simulink model "lander"  (R2016b)
settings: Solver=FixedStepDiscrete  StartTime=0.0  StopTime=10  FixedStep=0.1  RelTol=1e-3
undefined symbols (not defined in the file): AtmosphereDensityRate, DiscIntNeverNeededParam, GravityConstant, InitialHeight, InitialVelocity, Mass, ProcessNoise
settings Model: Creator=csax  LastModifiedBy=csax
settings OptimizationCC: DefaultParameterBehavior=Inlined
settings DebuggingCC: ParameterTunabilityLossMsg=error
settings HardwareCC: ProdBitPerPointer=32  ProdBitPerSizeT=32  ProdBitPerPtrDiffT=32  ProdLargestAtomicFloat=None  ProdWordSize=32  ProdHWDeviceType=Custom Processor->Custom
settings RTWCC: SystemTargetFile=trace32_target_ert.tlc  MakeCommand=trace32_target_make  TemplateMakefile=trace32_arm_tmf.tmf  Description=TRACE32 Target  GenerateReport=on  IncludeHyperlinkInReport=on  LaunchReport=on  GenerateTraceInfo=on  GenerateTraceReport=on  GenerateTraceReportSl=on  GenerateTraceReportSf=on  GenerateTraceReportEml=on
settings CodeAppCC: ForceParamTrailComments=on  IgnoreCustomStorageClasses=off  OperatorAnnotations=on  SimulinkDataObjDesc=on  SFDataObjDesc=on  MATLABFcnDesc=on  InsertBlockDesc=on  MATLABSourceComments=on
settings STFCustomTargetCC: TargetLangStandard=C99 (ISO)  CombineOutputUpdateFcns=on  ERTCustomFileBanners=on  SupportContinuousTime=off  SupportNonInlinedSFcns=off  RemoveResetFunc=on  MATLABClassNameForMDSCustomization=Simulink.SoftwareTarget.ERTCustomization  GRTInterface=off  SystemTargetFile=trace32_target_ert.tlc
settings ERTTargetCC: TargetLangStandard=C99 (ISO)  ParMdlRefBuildCompliant=off  CompOptLevelCompliant=off  ConcurrentExecutionCompliant=off  ERTFirstTimeCompliant=off  ModelStepFunctionPrototypeControlCompliant=off  CPPClassGenCompliant=off  UseToolchainInfoCompliant=off  InlinedParameterPlacement=NonHierarchical  ERTCustomFileTemplate=example_file_process.tlc

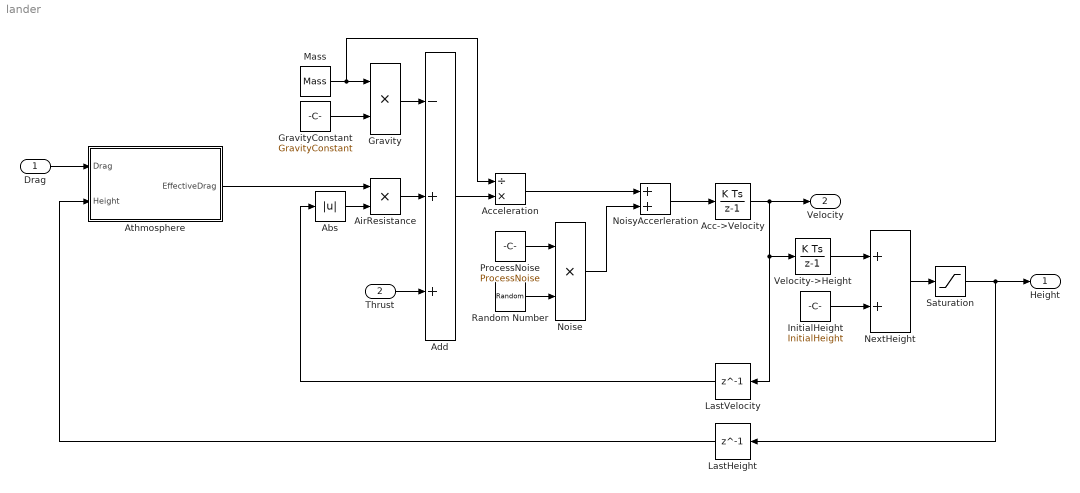
== system lander ==
  Drag : Inport
  Thrust : Inport  Port=2
  " InitialHeight" : Constant  Value=InitialHeight
  Abs : Abs
  Acc->Velocity : DiscreteIntegrator  InitialConditionSetting=State (most efficient)  SampleTime=-1  ICPrevOutput=DiscIntNeverNeededParam  ICPrevScaledInput=DiscIntNeverNeededParam
  Acceleration : Product  Inputs=/*
  Add : Sum  Inputs=-++
  AirResistance : Product
  Athmosphere : Subsystem
  Gravity : Product
  GravityConstant : Constant  Value=GravityConstant
  LastHeight : Delay  DelayLength=1  InitialCondition=InitialVelocity
  LastVelocity : Delay  DelayLength=1  InitialCondition=InitialVelocity
  Mass : Constant  Value=Mass
  NextHeight : Sum
  Noise : Product
  NoisyAccerleration : Sum
  ProcessNoise : Constant  Value=ProcessNoise
  Random Number : RandomNumber  SampleTime=0.1
  Saturation : Saturate  UpperLimit=Inf  LowerLimit=0
  Velocity->Height : DiscreteIntegrator  InitialConditionSetting=State (most efficient)  SampleTime=-1  ICPrevOutput=DiscIntNeverNeededParam  ICPrevScaledInput=DiscIntNeverNeededParam
  Height : Outport
  Velocity : Outport  Port=2
  wires:
  NoisyAccerleration/1 -> Acc->Velocity/1
  ProcessNoise/1 -> Noise/1
  Random Number/1 -> Noise/2
  NextHeight/1 -> Saturation/1
  Add/1 -> Acceleration/2
  Thrust/1 -> Add/3
  Acceleration/1 -> NoisyAccerleration/1
  GravityConstant/1 -> Gravity/2
  Mass/1 -> Acceleration/1, Gravity/1
  Acc->Velocity/1 -> LastVelocity/1, Velocity->Height/1, Velocity/1
  Athmosphere/1(EffectiveDrag) -> AirResistance/1
  LastVelocity/1 -> Abs/1
  Velocity->Height/1 -> NextHeight/1
  Gravity/1 -> Add/1
  Drag/1 -> Athmosphere/1(Drag)
  LastHeight/1 -> Athmosphere/2(Height)
  Saturation/1 -> LastHeight/1, Height/1
  Abs/1 -> AirResistance/2
  AirResistance/1 -> Add/2
  " InitialHeight"/1 -> NextHeight/2
  Noise/1 -> NoisyAccerleration/2

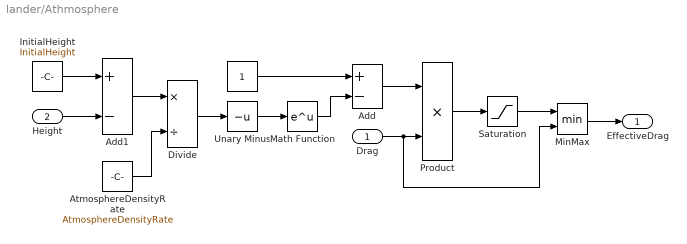
== system lander/Athmosphere ==
  Drag : Inport
  Height : Inport  Port=2
  " " : Constant
  " AtmosphereDensityRate" : Constant  Value=AtmosphereDensityRate
  " InitialHeight" : Constant  Value=InitialHeight
  Add : Sum  Inputs=+-
  Add1 : Sum  Inputs=+-
  Divide : Product  Inputs=*/
  Math Function : Math  SaturateOnIntegerOverflow=on
  MinMax : MinMax  Inputs=2
  Product : Product
  Saturation : Saturate  UpperLimit=+Inf  LowerLimit=0
  Unary Minus : UnaryMinus
  EffectiveDrag : Outport
  wires:
  " InitialHeight"/1 -> Add1/1
  " "/1 -> Add/1
  Height/1 -> Add1/2
  Add1/1 -> Divide/1
  " AtmosphereDensityRate"/1 -> Divide/2
  Add/1 -> Product/1
  Drag/1 -> MinMax/2, Product/2
  Math Function/1 -> Add/2
  Product/1 -> Saturation/1
  Divide/1 -> Unary Minus/1
  Unary Minus/1 -> Math Function/1
  Saturation/1 -> MinMax/1
  MinMax/1 -> EffectiveDrag/1
